simulink model "testsift"  (R2015a)
settings: Solver=ode45  StartTime=0.0  StopTime=10.0  RelTol=1e-3
InitFcn:
  | %% DSPBuilder Start
  | alt_dspbuilder_update_model(bdroot)
  | %% DSPBuilder End
libraries: allblocks_alteradspbuilder2 x2280
(part 1 of 26)
settings Model: Creator=ASUS  LastModifiedBy=ASUS

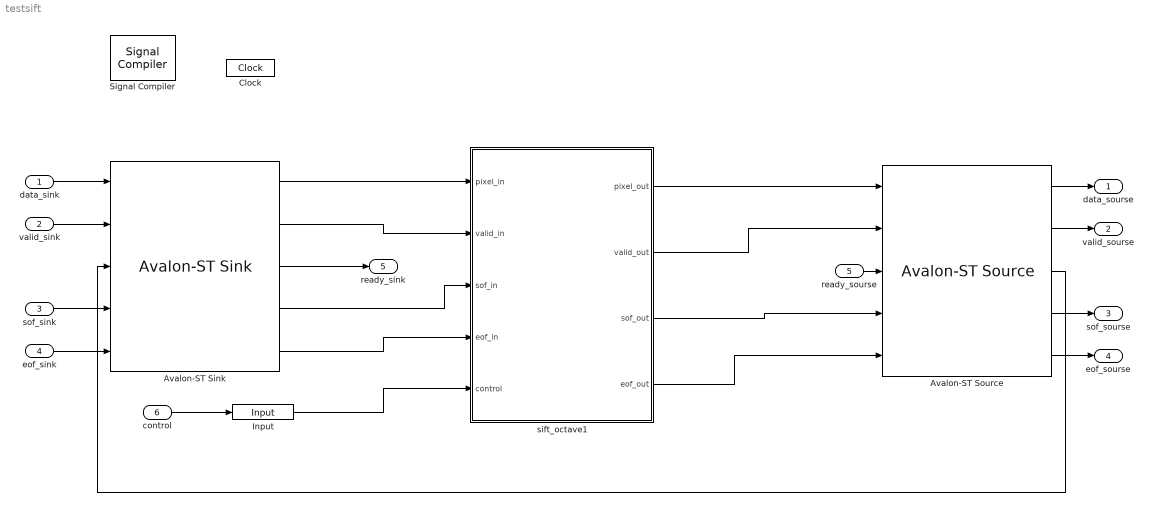
== system testsift ==
  data_sink : Inport
  valid_sink : Inport  Port=2
  sof_sink : Inport  Port=3
  eof_sink : Inport  Port=4
  ready_sourse : Inport  Port=5
  control : Inport  Port=6
  Avalon-ST Sink : allblocks_alteradspbuilder2/Avalon-ST Sink  iofile=C:\Users\ASUS\Desktop\sift_fpga\Octave_2\tb_testsift\testsift_Avalon-ST+Sink_data.salt,C:\Users\ASUS\Desktop\sift_fpga\Octave_2\tb_testsift\testsift_Avalon-ST+Sink_valid.salt,C:\Users\ASUS\Desktop\sift_fpga\Octave_2\tb_testsift\testsift_Avalon-ST+Sink_ready.capture,C:\Users\ASUS\Desktop\sift_fpga\Octave_2\tb_testsift\testsift_Avalon-ST+Sink_startofpacket.salt,C:\Users\ASUS\Desktop\sift_fpga\Octave_2\tb_testsift\testsift_Avalon-ST+Sink_endofpacket.salt,  SpecifyClock=off  BusType=Unsigned Integer  bwl=24  bwr=0  symbolWidth=8  symbolsPerBeat=3  numOfChannels=0  numOfErrorDescriptors=0  endOfPacket=on  startOfPacket=on  empty=off  readyLatency=1  externalType=Inferred  PORTTYPE=Output
  Avalon-ST Source : allblocks_alteradspbuilder2/Avalon-ST Source  iofile=C:\Users\ASUS\Desktop\sift_fpga\Octave_2\tb_testsift\testsift_Avalon-ST+Source_data.capture,C:\Users\ASUS\Desktop\sift_fpga\Octave_2\tb_testsift\testsift_Avalon-ST+Source_valid.capture,C:\Users\ASUS\Desktop\sift_fpga\Octave_2\tb_testsift\testsift_Avalon-ST+Source_ready.salt,C:\Users\ASUS\Desktop\sift_fpga\Octave_2\tb_testsift\testsift_Avalon-ST+Source_startofpacket.capture,C:\Users\ASUS\Desktop\sift_fpga\Octave_2\tb_testsift\testsift_Avalon-ST+Source_endofpacket.capture,  SpecifyClock=off  BusType=Unsigned Integer  bwl=24  bwr=0  symbolWidth=8  symbolsPerBeat=3  numOfChannels=0  numOfErrorDescriptors=0  endOfPacket=on  startOfPacket=on  empty=off  readyLatency=1  externalType=Inferred  PORTTYPE=Input
  Clock : allblocks_alteradspbuilder2/Clock  ClockPeriod=10/1.5  ClockPeriodUnit=ns  SampleTime=1  ResetLatency=0  ResetRegisterCascadeDepth=0  SimulationStartCycle=5  PhaseOffset=0  Reset=aclr  ResetType=Active Low  Export=off
  Input : allblocks_alteradspbuilder2/Input  iofile=C:\Users\ASUS\Desktop\sift_fpga\Octave_2\tb_testsift\testsift_Input.salt  BusType=Unsigned Integer  bwl=18  bwr=0  SpecifyClock=off  PORTTYPE=Input  externalType=Inferred  allowFloatingPointOverride=on  logOutputs=off
  Signal Compiler : allblocks_alteradspbuilder2/Signal Compiler  DeviceFamily=Cyclone IV GX  DeviceName=AUTO  DisableEarlyHDLGeneration=off  EnableSignalTap=off  SignalTapDepth=128  UseBoardBlock=off  StpUseDefaultClock=on  StpClock=Clock  ExportDir=C:\altera\16.0\quartus\dsp_builder  MAX10_ProgrammingMode=Internal Flash (SDM) Single Boot
  sift_octave1 : Subsystem
  data_sourse : Outport
  valid_sourse : Outport  Port=2
  sof_sourse : Outport  Port=3
  eof_sourse : Outport  Port=4
  ready_sink : Outport  Port=5
  wires:
  sift_octave1/1(pixel_out) -> Avalon-ST Source/1
  Avalon-ST Sink/1 -> sift_octave1/1(pixel_in)
  Avalon-ST Sink/2 -> sift_octave1/2(valid_in)
  sift_octave1/2(valid_out) -> Avalon-ST Source/2
  sift_octave1/3(sof_out) -> Avalon-ST Source/4
  sift_octave1/4(eof_out) -> Avalon-ST Source/5
  Avalon-ST Sink/5 -> sift_octave1/4(eof_in)
  Avalon-ST Sink/4 -> sift_octave1/3(sof_in)
  Avalon-ST Source/3 -> Avalon-ST Sink/3
  Avalon-ST Source/1 -> data_sourse/1
  Avalon-ST Source/2 -> valid_sourse/1
  Avalon-ST Source/4 -> sof_sourse/1
  Avalon-ST Source/5 -> eof_sourse/1
  data_sink/1 -> Avalon-ST Sink/1
  valid_sink/1 -> Avalon-ST Sink/2
  sof_sink/1 -> Avalon-ST Sink/4
  eof_sink/1 -> Avalon-ST Sink/5
  ready_sourse/1 -> Avalon-ST Source/3
  Avalon-ST Sink/3 -> ready_sink/1
  control/1 -> Input/1
  Input/1 -> sift_octave1/5(control)

== system testsift/sift_octave1 ==
  pixel_in : Inport
  valid_in : Inport  Port=2
  sof_in : Inport  Port=3
  eof_in : Inport  Port=4
  control : Inport  Port=5
  AltBus : allblocks_alteradspbuilder2/AltBus  BusType=Unsigned Integer  bwl=128  bwr=0  saturate=off  floatingPointInput=on  floatingPointOutput=on  logOutputs=off  logFile=C:\Users\ASUS\Desktop\sift_fpga\Octave_2\tb_testSiftOctave1\testSiftOctave1_sift%5Foctave1_AltBus.fixedpointlog
  AltBus1 : allblocks_alteradspbuilder2/AltBus  BusType=Unsigned Integer  bwl=1173  bwr=0  saturate=off  floatingPointInput=on  floatingPointOutput=on  logOutputs=off  logFile=C:\Users\ASUS\Desktop\sift_fpga\Octave_2\tb_testSiftOctave1\testSiftOctave1_sift%5Foctave1_AltBus1.fixedpointlog
  AltBus2 : allblocks_alteradspbuilder2/AltBus  BusType=Unsigned Integer  bwl=8  bwr=0  saturate=off  floatingPointInput=on  floatingPointOutput=on  logOutputs=off  logFile=C:\Users\ASUS\Desktop\sift_fpga\Octave_2\tb_testSiftOctave1\testSiftOctave1_sift%5Foctave1_AltBus2.fixedpointlog
  AltBus3 : allblocks_alteradspbuilder2/AltBus  BusType=Unsigned Integer  bwl=10  bwr=0  saturate=off  floatingPointInput=on  floatingPointOutput=on  logOutputs=off  logFile=C:\Users\ASUS\Desktop\sift_fpga\Octave_2\tb_testSiftOctave1\testSiftOctave1_sift%5Foctave1_AltBus3.fixedpointlog
  AltBus4 : allblocks_alteradspbuilder2/AltBus  BusType=Unsigned Integer  bwl=8  bwr=0  saturate=off  floatingPointInput=on  floatingPointOutput=on  logOutputs=off  logFile=C:\Users\ASUS\Desktop\sift_fpga\Octave_2\tb_testSiftOctave1\testSiftOctave1_sift%5Foctave1_AltBus4.fixedpointlog
  AltBus5 : allblocks_alteradspbuilder2/AltBus  BusType=Unsigned Integer  bwl=18  bwr=0  saturate=off  floatingPointInput=on  floatingPointOutput=on  logOutputs=off  logFile=C:\Users\ASUS\Desktop\sift_fpga\Octave_2\tb_testSiftOctave1\testSiftOctave1_sift%5Foctave1_AltBus5.fixedpointlog
  Bus_Concatenation : Subsystem
  GradOrien : Subsystem
  Line_buff_11x11 : Subsystem
  Memory Delay : allblocks_alteradspbuilder2/Memory Delay  BusType=Unsigned Integer  bwl=1  bwr=0  pipeline=4495  pipeline_display=4495  ram_type=AUTO  use_ena=on  use_sclr=off  allowFloatingPointOverride=on  logOutputs=off  logFile=C:\Users\ASUS\Desktop\sift_fpga\Octave_2\tb_testSiftOctave1\testSiftOctave1_sift%5Foctave1_Memory+Delay.fixedpointlog
  Memory Delay1 : allblocks_alteradspbuilder2/Memory Delay  BusType=Unsigned Integer  bwl=10  bwr=0  pipeline=6443  pipeline_display=6443  ram_type=AUTO  use_ena=on  use_sclr=off  allowFloatingPointOverride=on  logOutputs=off  logFile=C:\Users\ASUS\Desktop\sift_fpga\Octave_2\tb_testSiftOctave1\testSiftOctave1_sift%5Foctave1_Memory+Delay1.fixedpointlog
  Memory Delay2 : allblocks_alteradspbuilder2/Memory Delay  BusType=Unsigned Integer  bwl=10  bwr=0  pipeline=6443  pipeline_display=6443  ram_type=AUTO  use_ena=on  use_sclr=off  allowFloatingPointOverride=on  logOutputs=off  logFile=C:\Users\ASUS\Desktop\sift_fpga\Octave_2\tb_testSiftOctave1\testSiftOctave1_sift%5Foctave1_Memory+Delay2.fixedpointlog
  Memory Delay3 : allblocks_alteradspbuilder2/Memory Delay  BusType=Unsigned Integer  bwl=24  bwr=0  pipeline=6443  pipeline_display=6443  ram_type=AUTO  use_ena=on  use_sclr=off  allowFloatingPointOverride=on  logOutputs=off  logFile=C:\Users\ASUS\Desktop\sift_fpga\Octave_2\tb_testSiftOctave1\testSiftOctave1_sift%5Foctave1_Memory+Delay3.fixedpointlog
  Memory Delay4 : allblocks_alteradspbuilder2/Memory Delay  BusType=Unsigned Integer  bwl=1  bwr=0  pipeline=6443  pipeline_display=6443  ram_type=AUTO  use_ena=on  use_sclr=off  allowFloatingPointOverride=on  logOutputs=off  logFile=C:\Users\ASUS\Desktop\sift_fpga\Octave_2\tb_testSiftOctave1\testSiftOctave1_sift%5Foctave1_Memory+Delay4.fixedpointlog
  Memory Delay5 : allblocks_alteradspbuilder2/Memory Delay  BusType=Unsigned Integer  bwl=1  bwr=0  pipeline=6443  pipeline_display=6443  ram_type=AUTO  use_ena=on  use_sclr=off  allowFloatingPointOverride=on  logOutputs=off  logFile=C:\Users\ASUS\Desktop\sift_fpga\Octave_2\tb_testSiftOctave1\testSiftOctave1_sift%5Foctave1_Memory+Delay5.fixedpointlog
  calculate_key_point : Subsystem
  counter : Subsystem
  descriptor : Subsystem
  dog_space : Subsystem
  hist_bin : Subsystem
  matching : Subsystem
  scale_space : Subsystem
  pixel_out : Outport
  valid_out : Outport  Port=2
  sof_out : Outport  Port=3
  eof_out : Outport  Port=4
  wires:
  dog_space/2(dog2_out) -> calculate_key_point/2(pixel_dog2_in)
  dog_space/1(dog3_out) -> calculate_key_point/1(pixel_dog3_in)
  [valid_in] -> hist_bin/3(clken)
  GradOrien/2(orien) -> AltBus2/1
  [valid_in] -> scale_space/2(valid_in)
  [valid_in] -> GradOrien/2(clken)
  GradOrien/1(m_xy) -> AltBus3/1
  hist_bin/6(hist_bin6_out) -> Bus_Concatenation/6(bin6_in)
  scale_space/2(scale3) -> dog_space/2(scale3_in)
  scale_space/4(scale1) -> dog_space/4(scale1_in)
  [valid_in] -> calculate_key_point/4(valid_in)
  hist_bin/8(hist_bin8_out) -> Bus_Concatenation/8(bin8_in)
  scale_space/3(scale2) -> GradOrien/1(data_in), dog_space/3(scale2_in)
  scale_space/1(scale4) -> dog_space/1(scale4_in)
  [pixel_in] -> AltBus4/1
  [valid_in] -> dog_space/5(valid_in)
  Line_buff_11x11/5(Out55) -> descriptor/5(data_in55)
  Line_buff_11x11/1(Out00) -> descriptor/1(data_in00)
  Line_buff_11x11/7(Out100) -> descriptor/7(data_in100)
  hist_bin/4(hist_bin4_out) -> Bus_Concatenation/4(bin4_in)
  Memory Delay2/1 -> descriptor/12(row_in)
  eof_in/1 -> [eof_in]
  [row] -> Memory Delay2/1
  Line_buff_11x11/9(Out1010) -> descriptor/9(data_in1010)
  Bus_Concatenation/1(hist_bin) -> AltBus/1
  hist_bin/2(hist_bin2_out) -> Bus_Concatenation/2(bin2_in)
  Line_buff_11x11/8(Out105) -> descriptor/8(data_in105)
  sof_in/1 -> [sof_in]
  Line_buff_11x11/6(Out510) -> descriptor/6(data_in510)
  counter/1(col_out) -> [column]
  hist_bin/3(hist_bin3_out) -> Bus_Concatenation/3(biin3_in)
  hist_bin/5(hist_bin5_out) -> Bus_Concatenation/5(bin5_in)
  hist_bin/1(hist_bin1_out) -> Bus_Concatenation/1(bin1_in)
  [eof_in] -> counter/2(eof_in)
  [valid_in] -> counter/1(valid_in)
  [valid_in] -> Line_buff_11x11/2(clken)
  Memory Delay/1 -> descriptor/10(isKeyPoint_in)
  descriptor/1(descriptor_out) -> AltBus1/1
  dog_space/3(dog1_out) -> calculate_key_point/3(pixel_dog1_in)
  hist_bin/7(hist_bin7_out) -> Bus_Concatenation/7(bin_in)
  [column] -> Memory Delay1/1
  Line_buff_11x11/3(Out010) -> descriptor/3(data_in010)
  counter/2(row_out) -> [row]
  Memory Delay1/1 -> descriptor/11(column_in)
  calculate_key_point/1(is_KeyPoint) -> Memory Delay/1
  Line_buff_11x11/2(Out05) -> descriptor/2(data_in05)
  Line_buff_11x11/4(Out50) -> descriptor/4(data_in50)
  control/1 -> [control]
  matching/3(eof_out) -> [eof_out]
  pixel_in/1 -> [pixel_in]
  valid_in/1 -> [valid_in]
  AltBus1/1 -> matching/1(descriptor_in)
  [sof_out] -> sof_out/1
  [valid_in] -> Memory Delay/2, Memory Delay1/2, Memory Delay2/2
  [pixel_out] -> pixel_out/1
  AltBus2/1 -> hist_bin/2(orien_In)
  matching/1(pixel_out) -> [pixel_out]
  [valid_in] -> Memory Delay5/2, Memory Delay3/2, Memory Delay4/2, matching/6(valid_in)
  matching/4(valid_out) -> [valid_out]
  [valid_out] -> valid_out/1
  matching/2(sof_out) -> [sof_out]
  AltBus/1 -> Line_buff_11x11/1(dataIn)
  [control] -> AltBus5/1
  AltBus3/1 -> hist_bin/1(m_xy_In)
  [eof_out] -> eof_out/1
  AltBus4/1 -> scale_space/1(data_in)
  [pixel_in] -> Memory Delay3/1
  Memory Delay3/1 -> matching/3(pixel_in)
  Memory Delay4/1 -> matching/4(eof_in)
  [eof_in] -> Memory Delay4/1
  Memory Delay5/1 -> matching/5(sof_in)
  [sof_in] -> Memory Delay5/1
  AltBus5/1 -> matching/2(control)

== system testsift/sift_octave1/Bus_Concatenation ==
  bin1_in : Inport
  bin2_in : Inport  Port=2
  biin3_in : Inport  Port=3
  bin4_in : Inport  Port=4
  bin5_in : Inport  Port=5
  bin6_in : Inport  Port=6
  bin_in : Inport  Port=7
  bin8_in : Inport  Port=8
  Bus Concatenation{,1..3} (4 alike) : allblocks_alteradspbuilder2/Bus Concatenation  isSigned=off  awidth=16  bwidth=16  pipeline_display=0
  Bus Concatenation7 : allblocks_alteradspbuilder2/Bus Concatenation  isSigned=off  awidth=32  bwidth=32  pipeline_display=0
  Bus Concatenation8 : allblocks_alteradspbuilder2/Bus Concatenation  isSigned=off  awidth=32  bwidth=32  pipeline_display=0
  Bus Concatenation9 : allblocks_alteradspbuilder2/Bus Concatenation  isSigned=off  awidth=64  bwidth=64  pipeline_display=0
  hist_bin : Outport
  wires:
  bin1_in/1 -> [bin1]
  bin2_in/1 -> [bin2]
  biin3_in/1 -> [bin3]
  bin4_in/1 -> [bin4]
  bin5_in/1 -> [bin5]
  bin6_in/1 -> [bin6]
  bin_in/1 -> [bin7]
  bin8_in/1 -> [bin8]
  Bus Concatenation/1 -> Bus Concatenation8/2
  [bin6] -> Bus Concatenation1/2
  Bus Concatenation1/1 -> Bus Concatenation8/1
  [bin8] -> Bus Concatenation/2
  [bin5] -> Bus Concatenation1/1
  [bin7] -> Bus Concatenation/1
  Bus Concatenation9/1 -> hist_bin/1
  [bin4] -> Bus Concatenation2/2
  [bin3] -> Bus Concatenation2/1
  [bin2] -> Bus Concatenation3/2
  [bin1] -> Bus Concatenation3/1
  Bus Concatenation3/1 -> Bus Concatenation7/1
  Bus Concatenation2/1 -> Bus Concatenation7/2
  Bus Concatenation7/1 -> Bus Concatenation9/1
  Bus Concatenation8/1 -> Bus Concatenation9/2

== system testsift/sift_octave1/GradOrien ==
  data_in : Inport
  clken : Inport  Port=2
  lineBuff_3x3 : Subsystem
  sub_GradOrian : Subsystem
  m_xy : Outport
  orien : Outport  Port=2
  wires:
  sub_GradOrian/1(orien) -> orien/1
  clken/1 -> sub_GradOrian/5(clken), lineBuff_3x3/2(clken)
  data_in/1 -> lineBuff_3x3/1(dataIn)
  sub_GradOrian/2(m_xy) -> m_xy/1
  lineBuff_3x3/1(Out01) -> sub_GradOrian/1(L_y_add_1)
  lineBuff_3x3/4(Out21) -> sub_GradOrian/4(L_y_sub_1)
  lineBuff_3x3/3(Out12) -> sub_GradOrian/3(L_x_sub_1)
  lineBuff_3x3/2(Out10) -> sub_GradOrian/2(L_x_add_1)

== system testsift/sift_octave1/Line_buff_11x11 ==
  dataIn : Inport
  clken : Inport  Port=2
  Memory Delay1 : allblocks_alteradspbuilder2/Memory Delay  BusType=Unsigned Integer  bwl=128  bwr=0  pipeline=1  pipeline_display=1  ram_type=AUTO  use_ena=on  use_sclr=off  allowFloatingPointOverride=on  logOutputs=off  logFile=C:\Users\ASUS\Desktop\sift_fpga\Octave_2\tb_testSiftOctave1\testSiftOctave1_sift%5Foctave1_Line%5Fbuff%5F11x11_Memory+Delay1.fixedpointlog
  Memory Delay11 : allblocks_alteradspbuilder2/Memory Delay  BusType=Unsigned Integer  bwl=128  bwr=0  pipeline=630  pipeline_display=630  ram_type=AUTO  use_ena=on  use_sclr=off  allowFloatingPointOverride=on  logOutputs=off  logFile=C:\Users\ASUS\Desktop\sift_fpga\Octave_2\tb_testSiftOctave1\testSiftOctave1_sift%5Foctave1_Line%5Fbuff%5F11x11_Memory+Delay11.fixedpointlog
  Memory Delay12 : allblocks_alteradspbuilder2/Memory Delay  BusType=Unsigned Integer  bwl=128  bwr=0  pipeline=5  pipeline_display=5  ram_type=AUTO  use_ena=on  use_sclr=off  allowFloatingPointOverride=on  logOutputs=off  logFile=C:\Users\ASUS\Desktop\sift_fpga\Octave_2\tb_testSiftOctave1\testSiftOctave1_sift%5Foctave1_Line%5Fbuff%5F11x11_Memory+Delay12.fixedpointlog
  Memory Delay13 : allblocks_alteradspbuilder2/Memory Delay  BusType=Unsigned Integer  bwl=128  bwr=0  pipeline=5  pipeline_display=5  ram_type=AUTO  use_ena=on  use_sclr=off  allowFloatingPointOverride=on  logOutputs=off  logFile=C:\Users\ASUS\Desktop\sift_fpga\Octave_2\tb_testSiftOctave1\testSiftOctave1_sift%5Foctave1_Line%5Fbuff%5F11x11_Memory+Delay13.fixedpointlog
  Memory Delay15 : allblocks_alteradspbuilder2/Memory Delay  BusType=Unsigned Integer  bwl=128  bwr=0  pipeline=630  pipeline_display=630  ram_type=AUTO  use_ena=on  use_sclr=off  allowFloatingPointOverride=on  logOutputs=off  logFile=C:\Users\ASUS\Desktop\sift_fpga\Octave_2\tb_testSiftOctave1\testSiftOctave1_sift%5Foctave1_Line%5Fbuff%5F11x11_Memory+Delay15.fixedpointlog
  Memory Delay16 : allblocks_alteradspbuilder2/Memory Delay  BusType=Unsigned Integer  bwl=128  bwr=0  pipeline=5  pipeline_display=5  ram_type=AUTO  use_ena=on  use_sclr=off  allowFloatingPointOverride=on  logOutputs=off  logFile=C:\Users\ASUS\Desktop\sift_fpga\Octave_2\tb_testSiftOctave1\testSiftOctave1_sift%5Foctave1_Line%5Fbuff%5F11x11_Memory+Delay16.fixedpointlog
  Memory Delay17 : allblocks_alteradspbuilder2/Memory Delay  BusType=Unsigned Integer  bwl=128  bwr=0  pipeline=5  pipeline_display=5  ram_type=AUTO  use_ena=on  use_sclr=off  allowFloatingPointOverride=on  logOutputs=off  logFile=C:\Users\ASUS\Desktop\sift_fpga\Octave_2\tb_testSiftOctave1\testSiftOctave1_sift%5Foctave1_Line%5Fbuff%5F11x11_Memory+Delay17.fixedpointlog
  Memory Delay18 : allblocks_alteradspbuilder2/Memory Delay  BusType=Unsigned Integer  bwl=128  bwr=0  pipeline=640*4  pipeline_display=2560  ram_type=AUTO  use_ena=on  use_sclr=off  allowFloatingPointOverride=on  logOutputs=off  logFile=C:\Users\ASUS\Desktop\sift_fpga\Octave_2\tb_testSiftOctave1\testSiftOctave1_sift%5Foctave1_Line%5Fbuff%5F11x11_Memory+Delay18.fixedpointlog
  Memory Delay5 : allblocks_alteradspbuilder2/Memory Delay  BusType=Unsigned Integer  bwl=128  bwr=0  pipeline=5  pipeline_display=5  ram_type=AUTO  use_ena=on  use_sclr=off  allowFloatingPointOverride=on  logOutputs=off  logFile=C:\Users\ASUS\Desktop\sift_fpga\Octave_2\tb_testSiftOctave1\testSiftOctave1_sift%5Foctave1_Line%5Fbuff%5F11x11_Memory+Delay5.fixedpointlog
  Memory Delay6 : allblocks_alteradspbuilder2/Memory Delay  BusType=Unsigned Integer  bwl=128  bwr=0  pipeline=5  pipeline_display=5  ram_type=AUTO  use_ena=on  use_sclr=off  allowFloatingPointOverride=on  logOutputs=off  logFile=C:\Users\ASUS\Desktop\sift_fpga\Octave_2\tb_testSiftOctave1\testSiftOctave1_sift%5Foctave1_Line%5Fbuff%5F11x11_Memory+Delay6.fixedpointlog
  Memory Delay7 : allblocks_alteradspbuilder2/Memory Delay  BusType=Unsigned Integer  bwl=128  bwr=0  pipeline=640*4  pipeline_display=2560  ram_type=AUTO  use_ena=on  use_sclr=off  allowFloatingPointOverride=on  logOutputs=off  logFile=C:\Users\ASUS\Desktop\sift_fpga\Octave_2\tb_testSiftOctave1\testSiftOctave1_sift%5Foctave1_Line%5Fbuff%5F11x11_Memory+Delay7.fixedpointlog
  Out00 : Outport
  Out05 : Outport  Port=2
  Out010 : Outport  Port=3
  Out50 : Outport  Port=4
  Out55 : Outport  Port=5
  Out510 : Outport  Port=6
  Out100 : Outport  Port=7
  Out105 : Outport  Port=8
  Out1010 : Outport  Port=9
  wires:
  [clken] -> Memory Delay11/2
  [clken] -> Memory Delay17/2
  [clken] -> Memory Delay6/2
  Memory Delay6/1 -> [data_010], Memory Delay7/1
  [clken] -> Memory Delay18/2
  Memory Delay18/1 -> Memory Delay15/1
  Memory Delay13/1 -> Memory Delay18/1, [data_510]
  [clken] -> Memory Delay15/2
  [clken] -> Memory Delay16/2
  Memory Delay17/1 -> [data_1010]
  Memory Delay16/1 -> Memory Delay17/1, [data_105]
  Memory Delay15/1 -> Memory Delay16/1, [data_100]
  [clken] -> Memory Delay7/2
  [clken] -> Memory Delay12/2
  Memory Delay11/1 -> Memory Delay12/1, [data_50]
  Memory Delay12/1 -> Memory Delay13/1, [data_55]
  Memory Delay7/1 -> Memory Delay11/1
  [clken] -> Memory Delay13/2
  [data_55] -> Out55/1
  [data_010] -> Out010/1
  [data_05] -> Out05/1
  clken/1 -> [clken]
  [data_00] -> Out00/1
  [data_50] -> Out50/1
  [data_100] -> Out100/1
  [data_510] -> Out510/1
  [data_1010] -> Out1010/1
  dataIn/1 -> [data_in]
  [data_105] -> Out105/1
  [clken] -> Memory Delay5/2
  Memory Delay1/1 -> Memory Delay5/1, [data_00]
  [clken] -> Memory Delay1/2
  [data_in] -> Memory Delay1/1
  Memory Delay5/1 -> Memory Delay6/1, [data_05]

== system testsift/sift_octave1/calculate_key_point ==
  pixel_dog3_in : Inport
  pixel_dog2_in : Inport  Port=2
  pixel_dog1_in : Inport  Port=3
  valid_in : Inport  Port=4
  AltBus : allblocks_alteradspbuilder2/AltBus  BusType=Signed Integer  bwl=9  bwr=0  saturate=off  floatingPointInput=on  floatingPointOutput=on  logOutputs=off  logFile=C:\Users\ASUS\Desktop\sift_fpga\Octave_2\tb_testSiftOctave1\testSiftOctave1_sift%5Foctave1_calculate%5Fkey%5Fpoint_AltBus.fixedpointlog
  AltBus1 : allblocks_alteradspbuilder2/AltBus  BusType=Signed Integer  bwl=9  bwr=0  saturate=off  floatingPointInput=on  floatingPointOutput=on  logOutputs=off  logFile=C:\Users\ASUS\Desktop\sift_fpga\Octave_2\tb_testSiftOctave1\testSiftOctave1_sift%5Foctave1_calculate%5Fkey%5Fpoint_AltBus1.fixedpointlog
  AltBus2 : allblocks_alteradspbuilder2/AltBus  BusType=Signed Integer  bwl=9  bwr=0  saturate=off  floatingPointInput=on  floatingPointOutput=on  logOutputs=off  logFile=C:\Users\ASUS\Desktop\sift_fpga\Octave_2\tb_testSiftOctave1\testSiftOctave1_sift%5Foctave1_calculate%5Fkey%5Fpoint_AltBus2.fixedpointlog
  find_KeyPoint : Subsystem
  line_buff_3x3 : Subsystem
  line_buff_3x3(1) : Subsystem
  line_buff_3x3(2) : Subsystem
  is_KeyPoint : Outport
  wires:
  line_buff_3x3/3(Out02) -> find_KeyPoint/3(dataIn_12)
  line_buff_3x3/6(Out12) -> find_KeyPoint/6(dataIn_15)
  line_buff_3x3/4(Out10) -> find_KeyPoint/4(dataIn_13)
  line_buff_3x3/5(Out11) -> find_KeyPoint/5(dataIn_14)
  line_buff_3x3(1)/2(Out01) -> find_KeyPoint/11(dataIn_21)
  line_buff_3x3(1)/3(Out02) -> find_KeyPoint/12(dataIn_22)
  line_buff_3x3(1)/4(Out10) -> find_KeyPoint/13(dataIn_23)
  line_buff_3x3/2(Out01) -> find_KeyPoint/2(dataIn_11)
  line_buff_3x3(2)/8(Out21) -> find_KeyPoint/26(dataIn_37)
  line_buff_3x3/8(Out21) -> find_KeyPoint/8(dataIn_17)
  line_buff_3x3/1(Out00) -> find_KeyPoint/1(dataIn_10)
  line_buff_3x3/7(Out20) -> find_KeyPoint/7(dataIn_16)
  line_buff_3x3/9(Out22) -> find_KeyPoint/9(dataIn_18)
  line_buff_3x3(1)/1(Out00) -> find_KeyPoint/10(dataIn_20)
  line_buff_3x3(2)/7(Out20) -> find_KeyPoint/25(dataIn_36)
  [pixel_dog2_in] -> AltBus1/1
  [pixel_dog1_in] -> AltBus/1
  [valid_in] -> line_buff_3x3(2)/2(clken)
  valid_in/1 -> [valid_in]
  [valid_in] -> line_buff_3x3(1)/2(clken)
  pixel_dog2_in/1 -> [pixel_dog2_in]
  pixel_dog1_in/1 -> [pixel_dog1_in]
  pixel_dog3_in/1 -> [pixel_dog3_in]
  [valid_in] -> line_buff_3x3/2(clken)
  [pixel_dog3_in] -> AltBus2/1
  line_buff_3x3(2)/2(Out01) -> find_KeyPoint/20(dataIn_31)
  line_buff_3x3(2)/3(Out02) -> find_KeyPoint/21(dataIn_32)
  line_buff_3x3(2)/4(Out10) -> find_KeyPoint/22(dataIn_33)
  line_buff_3x3(2)/5(Out11) -> find_KeyPoint/23(dataIn_34)
  line_buff_3x3(2)/1(Out00) -> find_KeyPoint/19(dataIn_30)
  line_buff_3x3(1)/5(Out11) -> find_KeyPoint/14(dataIn_24)
  line_buff_3x3(1)/6(Out12) -> find_KeyPoint/15(dataIn_25)
  line_buff_3x3(1)/7(Out20) -> find_KeyPoint/16(dataIn_26)
  line_buff_3x3(1)/8(Out21) -> find_KeyPoint/17(dataIn_27)
  line_buff_3x3(2)/6(Out12) -> find_KeyPoint/24(dataIn_35)
  line_buff_3x3(2)/9(Out22) -> find_KeyPoint/27(dataIn_38)
  line_buff_3x3(1)/9(Out22) -> find_KeyPoint/18(dataIn_28)
  find_KeyPoint/1(is_KeyPoint) -> is_KeyPoint/1
  AltBus/1 -> line_buff_3x3/1(dataIn)
  AltBus1/1 -> line_buff_3x3(1)/1(dataIn)
  AltBus2/1 -> line_buff_3x3(2)/1(dataIn)

== system testsift/sift_octave1/counter ==
  valid_in : Inport
  eof_in : Inport  Port=2
  Comparator : allblocks_alteradspbuilder2/Comparator  direction=a == b  pipeline_display=0  allowFloatingPointOverride=on  logOutputs=off  logFile=C:\Users\ASUS\Desktop\sift_fpga\Octave_2\tb_testSiftOctave1\testSiftOctave1_sift%5Foctave1_counter_Comparator.fixedpointlog
  Constant : allblocks_alteradspbuilder2/Constant  mask_cst=639  BusType=Unsigned Integer  bwl=10  bwr=0  roundMode=Truncate  satMode=Wrap  SpecifyClock=off  allowFloatingPointOverride=on  logOutputs=off  logFile=C:\Users\ASUS\Desktop\sift_fpga\Octave_2\tb_testSiftOctave1\testSiftOctave1_sift%5Foctave1_counter_Constant.fixedpointlog
  Counter : allblocks_alteradspbuilder2/Counter  BusType=Unsigned Integer  bwl=10  bwr=0  use_modulo=on  modulo=640  SpecifyClock=off  direction=Increment  use_sload=off  use_sset=off  svalue=1  use_clk_ena=off  use_ena=on  use_sclr=on  pipeline_display=1
  Counter1 : allblocks_alteradspbuilder2/Counter  BusType=Unsigned Integer  bwl=10  bwr=0  use_modulo=on  modulo=480  SpecifyClock=off  direction=Increment  use_sload=off  use_sset=off  svalue=0  use_clk_ena=off  use_ena=on  use_sclr=on  pipeline_display=1
  Logical Bit Operator : allblocks_alteradspbuilder2/Logical Bit Operator  LogicalOperator=AND  user_inputs=2  pipeline_display=0
  col_out : Outport
  row_out : Outport  Port=2
  wires:
  [eof_in] -> Counter1/2
  Logical Bit Operator/1 -> Counter1/1
  [counter_col] -> Comparator/1
  eof_in/1 -> [eof_in]
  Constant/1 -> Comparator/2
  Comparator/1 -> Logical Bit Operator/2
  valid_in/1 -> [valid_in]
  Counter1/1 -> [counter_row]
  Counter/1 -> [counter_col]
  [valid_in] -> Logical Bit Operator/1, Counter/1
  [counter_row] -> row_out/1
  [counter_col] -> col_out/1
  [eof_in] -> Counter/2

== system testsift/sift_octave1/descriptor ==
  data_in00 : Inport
  data_in05 : Inport  Port=2
  data_in010 : Inport  Port=3
  data_in50 : Inport  Port=4
  data_in55 : Inport  Port=5
  data_in510 : Inport  Port=6
  data_in100 : Inport  Port=7
  data_in105 : Inport  Port=8
  data_in1010 : Inport  Port=9
  isKeyPoint_in : Inport  Port=10
  column_in : Inport  Port=11
  row_in : Inport  Port=12
  AltBus : allblocks_alteradspbuilder2/AltBus  BusType=Unsigned Integer  bwl=128*9  bwr=0  saturate=off  floatingPointInput=on  floatingPointOutput=on  logOutputs=off  logFile=C:\Users\ASUS\Desktop\sift_fpga\Octave_2\tb_testSiftOctave1\testSiftOctave1_sift%5Foctave1_descriptor_AltBus.fixedpointlog
  AltBus1 : allblocks_alteradspbuilder2/AltBus  BusType=Single Bit  bwl=1  bwr=0  saturate=off  floatingPointInput=on  floatingPointOutput=on  logOutputs=off  logFile=C:\Users\ASUS\Desktop\sift_fpga\Octave_2\tb_testSiftOctave1\testSiftOctave1_sift%5Foctave1_descriptor_AltBus1.fixedpointlog
  AltBus2 : allblocks_alteradspbuilder2/AltBus  BusType=Single Bit  bwl=1  bwr=0  saturate=off  floatingPointInput=on  floatingPointOutput=on  logOutputs=off  logFile=C:\Users\ASUS\Desktop\sift_fpga\Octave_2\tb_testSiftOctave1\testSiftOctave1_sift%5Foctave1_descriptor_AltBus2.fixedpointlog
  AltBus3 : allblocks_alteradspbuilder2/AltBus  BusType=Unsigned Integer  bwl=10  bwr=0  saturate=off  floatingPointInput=on  floatingPointOutput=on  logOutputs=off  logFile=C:\Users\ASUS\Desktop\sift_fpga\Octave_2\tb_testSiftOctave1\testSiftOctave1_sift%5Foctave1_descriptor_AltBus3.fixedpointlog
  AltBus4 : allblocks_alteradspbuilder2/AltBus  BusType=Unsigned Integer  bwl=10  bwr=0  saturate=off  floatingPointInput=on  floatingPointOutput=on  logOutputs=off  logFile=C:\Users\ASUS\Desktop\sift_fpga\Octave_2\tb_testSiftOctave1\testSiftOctave1_sift%5Foctave1_descriptor_AltBus4.fixedpointlog
  Bus Concatenation : allblocks_alteradspbuilder2/Bus Concatenation  isSigned=off  awidth=1  bwidth=10  pipeline_display=0
  Bus Concatenation1 : allblocks_alteradspbuilder2/Bus Concatenation  isSigned=off  awidth=10  bwidth=128*9  pipeline_display=0
  Bus Concatenation2 : allblocks_alteradspbuilder2/Bus Concatenation  isSigned=off  awidth=11  bwidth=1162  pipeline_display=0
  BusSplitter : Subsystem
  Constant : allblocks_alteradspbuilder2/Constant  mask_cst=0  BusType=Unsigned Integer  bwl=1173  bwr=0  roundMode=Truncate  satMode=Wrap  SpecifyClock=off  allowFloatingPointOverride=on  logOutputs=off  logFile=C:\Users\ASUS\Desktop\sift_fpga\Octave_2\tb_testSiftOctave1\testSiftOctave1_sift%5Foctave1_descriptor_Constant.fixedpointlog
  Multiplexer : allblocks_alteradspbuilder2/Multiplexer  numInputs=2  pipeline=0  oneHot=off  pipeline_display=0  use_ena=off  use_aclr=off  allowFloatingPointOverride=on  logOutputs=off  logFile=C:\Users\ASUS\Desktop\sift_fpga\Octave_2\tb_testSiftOctave1\testSiftOctave1_sift%5Foctave1_descriptor_Multiplexer.fixedpointlog
  Multiplexer3 : allblocks_alteradspbuilder2/Multiplexer  numInputs=8  pipeline=0  oneHot=off  pipeline_display=0  use_ena=off  use_aclr=off  allowFloatingPointOverride=on  logOutputs=off  logFile=C:\Users\ASUS\Desktop\sift_fpga\Octave_2\tb_testSiftOctave1\testSiftOctave1_sift%5Foctave1_descriptor_Multiplexer3.fixedpointlog
  descriptor : Subsystem
  findMax : Subsystem
  descriptor_out : Outport
  wires:
  [hist_105] -> descriptor/8(data_in8)
  [hist_100] -> descriptor/7(data_in7)
  [hist_510] -> descriptor/6(data_in6)
  [hist_55] -> descriptor/5(data_in5)
  Multiplexer3/1 -> AltBus/1
  [hist_1010] -> descriptor/9(data_in9)
  descriptor/1(descriptor1) -> Multiplexer3/2
  [hist_05] -> descriptor/2(data_in2)
  [hist_010] -> descriptor/3(data_in3)
  [hist_50] -> descriptor/4(data_in4)
  descriptor/5(descriptor5) -> Multiplexer3/6
  descriptor/4(descriptor4) -> Multiplexer3/5
  [hist_00] -> descriptor/1(data_in1)
  descriptor/7(descriptor7) -> Multiplexer3/8
  descriptor/8(descriptor8) -> Multiplexer3/9
  descriptor/2(descriptor2) -> Multiplexer3/3
  descriptor/3(descriptor3) -> Multiplexer3/4
  descriptor/6(descriptor6) -> Multiplexer3/7
  BusSplitter/3(bin3) -> findMax/3(bin3)
  data_in00/1 -> [hist_00]
  data_in50/1 -> [hist_50]
  BusSplitter/1(bin1) -> findMax/1(bin1)
  data_in100/1 -> [hist_100]
  data_in010/1 -> [hist_010]
  data_in105/1 -> [hist_105]
  [hist_55] -> BusSplitter/1(data_in)
  data_in510/1 -> [hist_510]
  column_in/1 -> [column]
  data_in1010/1 -> [hist_1010]
  BusSplitter/8(bin8) -> findMax/8(bin8)
  data_in55/1 -> [hist_55]
  isKeyPoint_in/1 -> [isKeyPoint]
  row_in/1 -> [row]
  BusSplitter/4(bin4) -> findMax/4(bin4)
  BusSplitter/2(bin2) -> findMax/2(bin2)
  data_in05/1 -> [hist_05]
  BusSplitter/5(bin5) -> findMax/5(bin5)
  BusSplitter/7(bin7) -> findMax/7(bin7)
  BusSplitter/6(bin6) -> findMax/6(bin6)
  AltBus/1 -> [descriptor]
  [isKeyPoint] -> AltBus1/1
  Bus Concatenation/1 -> Bus Concatenation2/1
  Bus Concatenation1/1 -> Bus Concatenation2/2
  Bus Concatenation2/1 -> [descriptor_final]
  [isKeyPoint] -> AltBus2/1
  AltBus2/1 -> Multiplexer/1
  [descriptor_final] -> Multiplexer/3
  Constant/1 -> Multiplexer/2
  Multiplexer/1 -> descriptor_out/1
  AltBus1/1 -> Bus Concatenation/1
  findMax/1(bin_max) -> Multiplexer3/1
  [descriptor] -> Bus Concatenation1/2
  [column] -> AltBus3/1
  AltBus3/1 -> Bus Concatenation/2
  [row] -> AltBus4/1
  AltBus4/1 -> Bus Concatenation1/1

== system testsift/sift_octave1/dog_space ==
  scale4_in : Inport
  scale3_in : Inport  Port=2
  scale2_in : Inport  Port=3
  scale1_in : Inport  Port=4
  valid_in : Inport  Port=5
  Parallel Adder Subtractor : allblocks_alteradspbuilder2/Parallel Adder Subtractor  number_of_inputs=2  direction=+-  use_pipeline=on  pipeline_display=1  phase_selection=1  use_ena=on  use_aclr=off  allowFloatingPointOverride=on  logOutputs=off  logFile=C:\Users\ASUS\Desktop\sift_fpga\Octave_2\tb_testSiftOctave1\testSiftOctave1_sift%5Foctave1_dog%5Fspace_Parallel+Adder+Subtractor.fixedpointlog
  Parallel Adder Subtractor1 : allblocks_alteradspbuilder2/Parallel Adder Subtractor  number_of_inputs=2  direction=+-  use_pipeline=on  pipeline_display=1  phase_selection=1  use_ena=on  use_aclr=off  allowFloatingPointOverride=on  logOutputs=off  logFile=C:\Users\ASUS\Desktop\sift_fpga\Octave_2\tb_testSiftOctave1\testSiftOctave1_sift%5Foctave1_dog%5Fspace_Parallel+Adder+Subtractor1.fixedpointlog
  Parallel Adder Subtractor2 : allblocks_alteradspbuilder2/Parallel Adder Subtractor  number_of_inputs=2  direction=+-  use_pipeline=on  pipeline_display=1  phase_selection=1  use_ena=on  use_aclr=off  allowFloatingPointOverride=on  logOutputs=off  logFile=C:\Users\ASUS\Desktop\sift_fpga\Octave_2\tb_testSiftOctave1\testSiftOctave1_sift%5Foctave1_dog%5Fspace_Parallel+Adder+Subtractor2.fixedpointlog
  dog3_out : Outport
  dog2_out : Outport  Port=2
  dog1_out : Outport  Port=3
  wires:
  [pixel_scale2] -> Parallel Adder Subtractor1/1
  Parallel Adder Subtractor1/1 -> dog1_out/1
  [pixel_scale3] -> Parallel Adder Subtractor/1
  [valid_in] -> Parallel Adder Subtractor2/3
  [pixel_scale2] -> Parallel Adder Subtractor/2
  [pixel_scale3] -> Parallel Adder Subtractor2/2
  Parallel Adder Subtractor/1 -> dog2_out/1
  [valid_in] -> Parallel Adder Subtractor1/3
  Parallel Adder Subtractor2/1 -> dog3_out/1
  [pixel_scale1] -> Parallel Adder Subtractor1/2
  [valid_in] -> Parallel Adder Subtractor/3
  [pixel_scale4] -> Parallel Adder Subtractor2/1
  scale4_in/1 -> [pixel_scale4]
  scale3_in/1 -> [pixel_scale3]
  scale2_in/1 -> [pixel_scale2]
  scale1_in/1 -> [pixel_scale1]
  valid_in/1 -> [valid_in]
